simulink model "robot_delta_PID_v3"  (R2024b)
settings: Solver=ode1  StartTime=0  StopTime=10  FixedStep=1e-6  MaxStep=1e-6  RelTol=1e-6
model workspace (MAT data in the model file):
  Ts = 1e-06
  kd1 = 14
  kd2 = 13.6
  kd3 = 37.9
  ki1 = 39
  ki2 = 36
  ki3 = 11.6
  kp1 = 12.6
  kp2 = 12.2
  kp3 = 14.4
undefined symbols (not defined in the file or in its folder): DiscIntNeverNeededParam
libraries: spsUniversalBridgeLib x6, spsCurrentMeasurementLib x6, spsDCVoltageSourceLib x3, spsStepperMotorLib x3, spspowerguiLib x1
settings Model: Creator=rodri  LastModifiedBy=rodri
settings SolverCC: InitialStep=1e-6

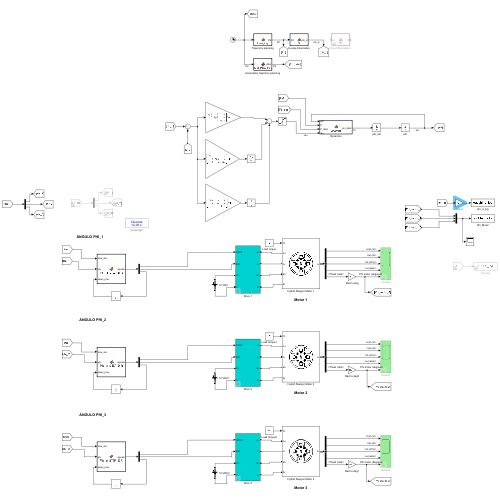
[thumbnail: Simulink's stored preview of the top-level diagram]
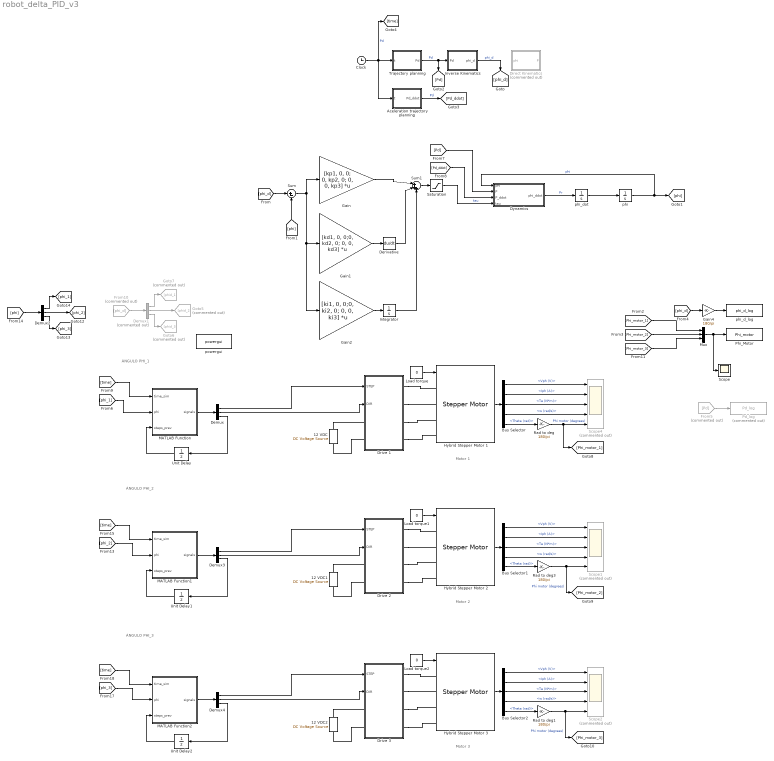
== system robot_delta_PID_v3 ==
  note: Motor 1
  note: ÁNGULO PHI_1
  note: ÁNGULO PHI_2
  note: ÁNGULO PHI_3
  note: Motor 2
  note: Motor 3
  12 VDC : spsDCVoltageSourceLib/DC Voltage Source  Amplitude=12  Measurements=None
  12 VDC1 : spsDCVoltageSourceLib/DC Voltage Source  Amplitude=12  Measurements=None
  12 VDC2 : spsDCVoltageSourceLib/DC Voltage Source  Amplitude=12  Measurements=None
  Aceleration trajectory planning : MATLAB Function  TreatAsAtomicUnit=on
  Bus Selector : BusSelector  OutputSignals=Vph (V),Iph (A),Te (N*m),w (rad/s),Theta (rad)
  Bus Selector1 : BusSelector  OutputSignals=Vph (V),Iph (A),Te (N*m),w (rad/s),Theta (rad)
  Bus Selector2 : BusSelector  OutputSignals=Vph (V),Iph (A),Te (N*m),w (rad/s),Theta (rad)
  Clock : Clock
  Demux{,2..4} (4 alike) : Demux  Outputs=3
  Demux1 : Demux  Commented=on  Outputs=3
  Derivative : Derivative
  Direct Kinematics : MATLAB Function  Commented=on  TreatAsAtomicUnit=on
  Drive 1 : Subsystem  mask{Iref=2, step=500, Ts=Ts}
      mask prompts: Iref "Phase current (A)"; step "Stepping rate (step/s)"; Ts "Sampling time (s)"
      mask init:
      | Nstep=round(1/step/Ts);
  Drive 2 : Subsystem  mask{Iref=2, step=500, Ts=Ts}
      mask prompts: Iref "Phase current (A)"; step "Stepping rate (step/s)"; Ts "Sampling time (s)"
      mask init:
      | Nstep=round(1/step/Ts);
  Drive 3 : Subsystem  mask{Iref=2, step=500, Ts=Ts}
      mask prompts: Iref "Phase current (A)"; step "Stepping rate (step/s)"; Ts "Sampling time (s)"
      mask init:
      | Nstep=round(1/step/Ts);
  Dynamics : MATLAB Function  TreatAsAtomicUnit=on
  From10 : From  Commented=on  GotoTag=phi_d
  From5 : From  Commented=on  GotoTag=Pd
  Gain : Gain  Gain=[kp1, 0, 0; 0, kp2, 0; 0, 0, kp3]  Multiplication=Matrix(K*u)
  Gain1 : Gain  Gain=[kd1, 0, 0;0, kd2, 0; 0, 0, kd3]  Multiplication=Matrix(K*u)
  Gain2 : Gain  Gain=[ki1, 0, 0;0, ki2, 0; 0, 0, ki3]  Multiplication=Matrix(K*u)
  Gain4 : Gain  Gain=180/pi
  Goto5 : Goto  Commented=on  GotoTag=phid_2
  Goto6 : Goto  Commented=on  GotoTag=phid_3
  Goto7 : Goto  Commented=on  GotoTag=phid_1
  Hybrid Stepper Motor 1 : spsStepperMotorLib/Stepper Motor  MotorType=Permanent-magnet / Hybrid  NumberOfPhases_1=2  NumberOfPhases_2=3  PresetModel_1=<empty>  PresetModel_2=<empty>  L=2.8e-3  Lmax=10e-3  Lmin=2e-3  R=1.5  Step_angle=360/1600  Psim=0.005  Tdm=2.2/100  J=54/(1000*100^2)  B=1e-7*1000  w0=0  pos0=0  TsPowergui=0  TsBlock=-1
  Hybrid Stepper Motor 2 : spsStepperMotorLib/Stepper Motor  MotorType=Permanent-magnet / Hybrid  NumberOfPhases_1=2  NumberOfPhases_2=3  PresetModel_1=<empty>  PresetModel_2=<empty>  L=2.8e-3  Lmax=10e-3  Lmin=2e-3  R=1.5  Step_angle=360/1600  Psim=0.005  Tdm=2.2/100  J=54/(1000*100^2)  B=1e-7*1000  w0=0  pos0=0  TsPowergui=0  TsBlock=-1
  Hybrid Stepper Motor 3 : spsStepperMotorLib/Stepper Motor  MotorType=Permanent-magnet / Hybrid  NumberOfPhases_1=2  NumberOfPhases_2=3  PresetModel_1=<empty>  PresetModel_2=<empty>  L=2.8e-3  Lmax=10e-3  Lmin=2e-3  R=1.5  Step_angle=360/1600  Psim=0.005  Tdm=2.2/100  J=54/(1000*100^2)  B=1e-7*1000  w0=0  pos0=0  TsPowergui=0  TsBlock=-1
  Integrator : Integrator  InitialCondition=[0;0;0]
  Inverse Kinematics : MATLAB Function  TreatAsAtomicUnit=on
  Load torque : Constant  Value=0
  Load torque1 : Constant  Value=0
  Load torque2 : Constant  Value=0
  MATLAB Function : MATLAB Function  TreatAsAtomicUnit=on
  MATLAB Function1 : MATLAB Function  TreatAsAtomicUnit=on
  MATLAB Function2 : MATLAB Function  TreatAsAtomicUnit=on
  Mux : Mux  Inputs=3
  Pd_log : ToWorkspace  Commented=on  VariableName=Pd_log  SampleTime=-1
  Phi_Motor : ToWorkspace  VariableName=Phi_motor  SampleTime=-1
  Rad to deg : Gain  Gain=180/pi
  Rad to deg1 : Gain  Gain=180/pi
  Rad to deg3 : Gain  Gain=180/pi
  Saturation : Saturate  UpperLimit=19.8  LowerLimit=-19.8
  Scope : Scope
  Scope1 : Scope  Commented=on  NumInputPorts=5
  Scope2 : Scope  Commented=on  NumInputPorts=5
  Scope4 : Scope  Commented=on  NumInputPorts=5
  Sum : Sum  Inputs=|+-
  Sum1 : Sum  Inputs=|+++
  Trajectory planning : MATLAB Function  TreatAsAtomicUnit=on
  Unit Delay : UnitDelay  SampleTime=-1  HasFrameUpgradeWarning=on
  Unit Delay1 : UnitDelay  SampleTime=-1  HasFrameUpgradeWarning=on
  Unit Delay2 : UnitDelay  SampleTime=-1  HasFrameUpgradeWarning=on
  phi : Integrator  InitialCondition=[0;0;0]
  phi_d_log : ToWorkspace  VariableName=phi_d_log  SampleTime=-1
  phi_dot : Integrator  InitialCondition=[0;0;0]
  powergui : spspowerguiLib/powergui  SimulationMode=Discrete  SampleTime=Ts  frequency=60  Iterations=50  frequencyindice=0  Pbase=100e6  ErrMax=1e-4  UnitsV=kV  UnitsW=MW  buscounter=0  FunctionMessages=off  echomessages=off  EnableUseOfTLC=off  CurrentSourceSwitches=off  DisableSnubberDevices=off  DisableRonSwitches=off  DisableVfSwitches=off  DisplayEquations=off  AutomaticDiscreteSolvers=off  SolverType=Tustin/Backward Euler (TBE)  Interpol=off  ExternalGateDelay=off  methode=off  Ts=0  x0status=blocks  SPID=off  SwTol=0  HookPort=off  NonlinearTolerance=1e-4  nMaxIteration=100  ContinueOnMaxIteration=off  RestoreLinks=warning  ResistiveCurrentMeasurement=off  Frange=[0:2:500]  Ylog=off  Xlog=on  ShowGrid=off  save=off  variable=ZData  structure=0  ZoomFFT=on  StartTime=0.0  cycles=1  DisplayStyle=1  fundamental=60  FreqAxis=off  MaxFrequency=1000  frequencyindicesteady=1  RmsSteady=1  display=off
  wires:
  Trajectory planning/1(Pd) -> Inverse Kinematics/1(Pd), [Pd]  "Pd"
  Inverse Kinematics/1(phi_d) -> [phi_d]  "phi_d"
  Dynamics/1(phi_ddot) -> phi_dot/1  "Pr"
  phi_dot/1 -> phi/1
  phi/1 -> Dynamics/1(phi), [phi]  "phi"
  [phi_d] -> Sum/1
  [phi] -> Sum/2
  Sum/1 -> Gain2/1, Gain1/1, Gain/1
  Gain1/1 -> Derivative/1
  Gain/1 -> Sum1/1
  Derivative/1 -> Sum1/2
  [Pd] -> Dynamics/2(P)
  [Pd_ddot] -> Dynamics/3(P_ddot)
  Clock/1 -> [time], Aceleration trajectory planning/1(t), Trajectory planning/1(t)  "Pd"
  Aceleration trajectory planning/1(Pd_ddot) -> [Pd_ddot]  "Pd"
  Gain2/1 -> Integrator/1
  Integrator/1 -> Sum1/3
  Sum1/1 -> Saturation/1
  Saturation/1 -> Dynamics/4(tau)  "tau"
  From5/1 -> Pd_log/1
  Demux2/2 -> [phi_2]
  Demux2/1 -> [phi_1]
  Demux2/3 -> [phi_3]
  [phi] -> Demux2/1
  [time] -> MATLAB Function/1(time_sim)
  Bus Selector/5 -> Rad to deg/1  "<Theta (rad)>"
  Hybrid Stepper Motor 1/1 -> Bus Selector/1
  Bus Selector/4 -> Scope4/4  "<w (rad/s)>"
  MATLAB Function/1(signals) -> Demux/1
  [phi_1] -> MATLAB Function/2(phi)
  Bus Selector/1 -> Scope4/1  "<Vph (V)>"
  Demux/1 -> Drive 1/1(STEP)
  Demux/2 -> Drive 1/2(DIR)
  Rad to deg/1 -> [Phi_motor_1], Scope4/5  "Phi motor (degrees)"
  Demux/3 -> Unit Delay/1
  Unit Delay/1 -> MATLAB Function/3(steps_prev)
  Bus Selector/2 -> Scope4/2  "<Iph (A)>"
  Bus Selector/3 -> Scope4/3  "<Te (N*m)>"
  Demux1/1 -> Goto7/1
  Demux1/3 -> Goto6/1
  From10/1 -> Demux1/1
  Demux1/2 -> Goto5/1
  Load torque/1 -> Hybrid Stepper Motor 1/1
  MATLAB Function1/1(signals) -> Demux3/1
  Demux3/1 -> Drive 2/1(STEP)
  Load torque1/1 -> Hybrid Stepper Motor 2/1
  Demux3/3 -> Unit Delay1/1
  Hybrid Stepper Motor 2/1 -> Bus Selector1/1
  Unit Delay1/1 -> MATLAB Function1/3(steps_prev)
  [time] -> MATLAB Function1/1(time_sim)
  [phi_2] -> MATLAB Function1/2(phi)
  Demux3/2 -> Drive 2/2(DIR)
  Bus Selector1/3 -> Scope1/3  "<Te (N*m)>"
  Rad to deg3/1 -> [Phi_motor_2], Scope1/5  "Phi motor (degrees)"
  Bus Selector1/4 -> Scope1/4  "<w (rad/s)>"
  Bus Selector1/2 -> Scope1/2  "<Iph (A)>"
  Bus Selector1/5 -> Rad to deg3/1  "<Theta (rad)>"
  Bus Selector1/1 -> Scope1/1  "<Vph (V)>"
  Bus Selector2/1 -> Scope2/1  "<Vph (V)>"
  Bus Selector2/2 -> Scope2/2  "<Iph (A)>"
  Rad to deg1/1 -> [Phi_motor_3], Scope2/5  "Phi motor (degrees)"
  [phi_3] -> MATLAB Function2/2(phi)
  Bus Selector2/3 -> Scope2/3  "<Te (N*m)>"
  Demux4/2 -> Drive 3/2(DIR)
  [time] -> MATLAB Function2/1(time_sim)
  Unit Delay2/1 -> MATLAB Function2/3(steps_prev)
  Hybrid Stepper Motor 3/1 -> Bus Selector2/1
  Demux4/3 -> Unit Delay2/1
  MATLAB Function2/1(signals) -> Demux4/1
  Demux4/1 -> Drive 3/1(STEP)
  Bus Selector2/5 -> Rad to deg1/1  "<Theta (rad)>"
  Bus Selector2/4 -> Scope2/4  "<w (rad/s)>"
  Load torque2/1 -> Hybrid Stepper Motor 3/1
  Mux/1 -> Scope/1, Phi_Motor/1
  Gain4/1 -> phi_d_log/1
  [phi_d] -> Gain4/1
  [Phi_motor_1] -> Mux/1
  [Phi_motor_2] -> Mux/2
  [Phi_motor_3] -> Mux/3
  connections:
  Drive 1/RConn3 -- Hybrid Stepper Motor 1/LConn3
  Drive 1/RConn4 -- Hybrid Stepper Motor 1/LConn4
  Drive 1/RConn2 -- Hybrid Stepper Motor 1/LConn2
  12 VDC/RConn1 -- Drive 1/LConn1
  Drive 1/LConn2 -- 12 VDC/LConn1
  Drive 1/RConn1 -- Hybrid Stepper Motor 1/LConn1
  12 VDC1/RConn1 -- Drive 2/LConn1
  Drive 2/RConn4 -- Hybrid Stepper Motor 2/LConn4
  Drive 2/LConn2 -- 12 VDC1/LConn1
  Drive 2/RConn1 -- Hybrid Stepper Motor 2/LConn1
  Drive 2/RConn2 -- Hybrid Stepper Motor 2/LConn2
  Drive 2/RConn3 -- Hybrid Stepper Motor 2/LConn3
  12 VDC2/RConn1 -- Drive 3/LConn1
  Drive 3/RConn4 -- Hybrid Stepper Motor 3/LConn4
  Drive 3/RConn1 -- Hybrid Stepper Motor 3/LConn1
  Drive 3/LConn2 -- 12 VDC2/LConn1
  Drive 3/RConn3 -- Hybrid Stepper Motor 3/LConn3
  Drive 3/RConn2 -- Hybrid Stepper Motor 3/LConn2

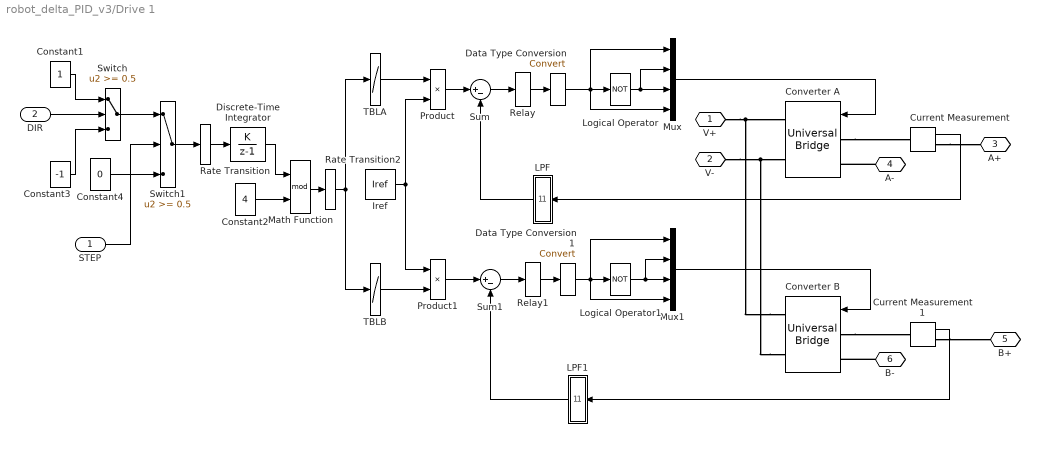
== system robot_delta_PID_v3/Drive 1 ==
  STEP : Inport
  DIR : Inport  Port=2
  Constant1 : Constant  SampleTime=Ts
  Constant2 : Constant  Value=4  SampleTime=Nstep*Ts
  Constant3 : Constant  Value=-1  SampleTime=Ts
  Constant4 : Constant  Value=0  SampleTime=Ts
  Converter A : spsUniversalBridgeLib/Universal Bridge  Arms=2  SnubberResistance=10000  SnubberCapacitance=inf  Device=MOSFET / Diodes  Ron=1e-3*10  Lon=0  ForwardVoltages="[  0  0  ]"  ForwardVoltage=0  GTOparameters=[ 10e-6 , 20e-6 ]  IGBTparameters=[ 0.5e-6 , 0.5e-6 ]  Measurements=None  Measurements_2=None  converterType=Rectifier
  Converter B : spsUniversalBridgeLib/Universal Bridge  Arms=2  SnubberResistance=10000  SnubberCapacitance=inf  Device=MOSFET / Diodes  Ron=1e-3*10  Lon=0  ForwardVoltages="[  0  0  ]"  ForwardVoltage=0  GTOparameters=[ 10e-6 , 20e-6 ]  IGBTparameters=[ 0.5e-6 , 0.5e-6 ]  Measurements=None  Measurements_2=None  converterType=Rectifier
  Current Measurement : spsCurrentMeasurementLib/Current Measurement  PhasorSimulation=off  OutputType=Complex  PSBequivalent=0
  Current Measurement1 : spsCurrentMeasurementLib/Current Measurement  PhasorSimulation=off  OutputType=Complex  PSBequivalent=0
  Data Type Conversion : DataTypeConversion  SaturateOnIntegerOverflow=off  RndMeth=Floor
  Data Type Conversion1 : DataTypeConversion  SaturateOnIntegerOverflow=off  RndMeth=Floor
  Discrete-Time Integrator : DiscreteIntegrator  IntegratorMethod=Accumulation: Forward Euler  SampleTime=Nstep*Ts  ICPrevOutput=DiscIntNeverNeededParam  ICPrevScaledInput=DiscIntNeverNeededParam
  Iref : Constant  Value=Iref  SampleTime=Ts
  LPF : Subsystem  mask{fc=10000, Ts=Ts}
      mask prompts: fc "Cut-off frequency (Hz)"; Ts "Sampling time (s)"
      mask init:
      | % fa=tf(1,[1/2/pi/fc 1]);
      | % fn=c2d(fa,Ts);
      | % [NN,DD]=tfdata(fn,'v')
      | 
      | NN = [ 0,0.0609];
      | DD = [1.0000,-0.9391];
  LPF1 : Subsystem  mask{fc=10000, Ts=Ts}
      mask prompts: fc "Cut-off frequency (Hz)"; Ts "Sampling time (s)"
      mask init:
      | % fa=tf(1,[1/2/pi/fc 1]);
      | % fn=c2d(fa,Ts);
      | % [NN,DD]=tfdata(fn,'v')
      | 
      | NN = [ 0,0.0609];
      | DD = [1.0000,-0.9391];
  Logical Operator : Logic  Operator=NOT  AllPortsSameDT=off  OutDataTypeStr=boolean
  Logical Operator1 : Logic  Operator=NOT  AllPortsSameDT=off  OutDataTypeStr=boolean
  Math Function : Math  Operator=mod  SignedPower=on  SampleTime=Nstep*Ts
  Mux : Mux
  Mux1 : Mux
  Product : Product  RndMeth=Zero
  Product1 : Product  RndMeth=Zero
  Rate Transition : RateTransition
  Rate Transition2 : RateTransition
  Relay : Relay  OnSwitchValue=0.01  OffSwitchValue=-0.01
  Relay1 : Relay  OnSwitchValue=0.01  OffSwitchValue=-0.01  OutDataTypeStr=Inherit: Inherit via back propagation
  Sum : Sum  Inputs=|+-  OutDataTypeStr=Inherit: Same as first input
  Sum1 : Sum  Inputs=|+-  OutDataTypeStr=Inherit: Same as first input
  Switch : Switch  Threshold=0.5  ZeroCross=off  SampleTime=Ts  SaturateOnIntegerOverflow=off  InputSameDT=off
  Switch1 : Switch  Threshold=0.5  ZeroCross=off  SampleTime=Ts  SaturateOnIntegerOverflow=off  InputSameDT=off
  TBLA : Lookup_n-D  NumberOfTableDimensions=1  BreakpointsForDimension1=[0:3]  BreakpointsForDimension2=[0 571.55 685.8 800.15 914.4 1028.8 1143.1 1257.4 1371.7 1486 1600.3 1714.6 1828.9 1943.2 2057.5 2171.8 2286.1 2400.5 2514.7 2629.1 2743.3 2857.7 2971.9 3086.3 3200.5 3314.9 3429.2]  Table=[1 0 -1 0]  InternalRulePriority=Speed  RndMeth=Simplest
  TBLB : Lookup_n-D  NumberOfTableDimensions=1  BreakpointsForDimension1=[0:3]  BreakpointsForDimension2=[0 571.55 685.8 800.15 914.4 1028.8 1143.1 1257.4 1371.7 1486 1600.3 1714.6 1828.9 1943.2 2057.5 2171.8 2286.1 2400.5 2514.7 2629.1 2743.3 2857.7 2971.9 3086.3 3200.5 3314.9 3429.2]  Table=[0 1 0 -1]  InternalRulePriority=Speed  RndMeth=Simplest
  V+ : PMIOPort  Side=Left
  V- : PMIOPort  Port=2  Side=Left
  A+ : PMIOPort  Port=3  Side=Right
  A- : PMIOPort  Port=4  Side=Right
  B+ : PMIOPort  Port=5  Side=Right
  B- : PMIOPort  Port=6  Side=Right
  wires:
  Constant4/1 -> Switch1/3
  Switch1/1 -> Rate Transition/1
  Switch/1 -> Switch1/1
  STEP/1 -> Switch1/2
  DIR/1 -> Switch/2
  Rate Transition2/1 -> TBLB/1, TBLA/1
  Math Function/1 -> Rate Transition2/1
  Product1/1 -> Sum1/1
  Product/1 -> Sum/1
  Rate Transition/1 -> Discrete-Time Integrator/1
  Constant3/1 -> Switch/3
  Constant1/1 -> Switch/1
  Discrete-Time Integrator/1 -> Math Function/1
  Constant2/1 -> Math Function/2
  Iref/1 -> Product1/1, Product/2
  TBLB/1 -> Product1/2
  TBLA/1 -> Product/1
  LPF1/1(O) -> Sum1/2
  LPF/1(O) -> Sum/2
  Data Type Conversion1/1 -> Mux1/4, Mux1/1, Logical Operator1/1
  Data Type Conversion/1 -> Logical Operator/1, Mux/4, Mux/1
  Current Measurement1/1 -> LPF1/1(I)
  Sum1/1 -> Relay1/1
  Mux1/1 -> Converter B/1
  Logical Operator1/1 -> Mux1/2, Mux1/3
  Relay1/1 -> Data Type Conversion1/1
  Mux/1 -> Converter A/1
  Logical Operator/1 -> Mux/2, Mux/3
  Relay/1 -> Data Type Conversion/1
  Current Measurement/1 -> LPF/1(I)
  Sum/1 -> Relay/1
  connections:
  Converter B/RConn2 -- Converter A/RConn2 -- V-/RConn1
  Converter B/RConn1 -- Converter A/RConn1 -- V+/RConn1
  Current Measurement1/RConn1 -- B+/RConn1
  Converter B/LConn1 -- Current Measurement1/LConn1
  Current Measurement/RConn1 -- A+/RConn1
  Converter A/LConn1 -- Current Measurement/LConn1
  B-/RConn1 -- Converter B/LConn2
  A-/RConn1 -- Converter A/LConn2

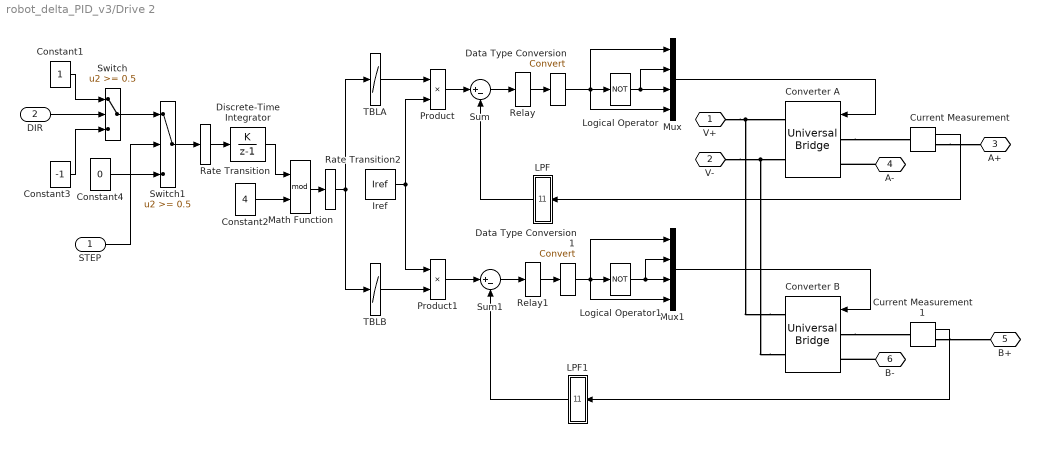
== system robot_delta_PID_v3/Drive 2 ==
  STEP : Inport
  DIR : Inport  Port=2
  Constant1 : Constant  SampleTime=Ts
  Constant2 : Constant  Value=4  SampleTime=Nstep*Ts
  Constant3 : Constant  Value=-1  SampleTime=Ts
  Constant4 : Constant  Value=0  SampleTime=Ts
  Converter A : spsUniversalBridgeLib/Universal Bridge  Arms=2  SnubberResistance=10000  SnubberCapacitance=inf  Device=MOSFET / Diodes  Ron=1e-3*10  Lon=0  ForwardVoltages="[  0  0  ]"  ForwardVoltage=0  GTOparameters=[ 10e-6 , 20e-6 ]  IGBTparameters=[ 0.5e-6 , 0.5e-6 ]  Measurements=None  Measurements_2=None  converterType=Rectifier
  Converter B : spsUniversalBridgeLib/Universal Bridge  Arms=2  SnubberResistance=10000  SnubberCapacitance=inf  Device=MOSFET / Diodes  Ron=1e-3*10  Lon=0  ForwardVoltages="[  0  0  ]"  ForwardVoltage=0  GTOparameters=[ 10e-6 , 20e-6 ]  IGBTparameters=[ 0.5e-6 , 0.5e-6 ]  Measurements=None  Measurements_2=None  converterType=Rectifier
  Current Measurement : spsCurrentMeasurementLib/Current Measurement  PhasorSimulation=off  OutputType=Complex  PSBequivalent=0
  Current Measurement1 : spsCurrentMeasurementLib/Current Measurement  PhasorSimulation=off  OutputType=Complex  PSBequivalent=0
  Data Type Conversion : DataTypeConversion  SaturateOnIntegerOverflow=off  RndMeth=Floor
  Data Type Conversion1 : DataTypeConversion  SaturateOnIntegerOverflow=off  RndMeth=Floor
  Discrete-Time Integrator : DiscreteIntegrator  IntegratorMethod=Accumulation: Forward Euler  SampleTime=Nstep*Ts  ICPrevOutput=DiscIntNeverNeededParam  ICPrevScaledInput=DiscIntNeverNeededParam
  Iref : Constant  Value=Iref  SampleTime=Ts
  LPF : Subsystem  mask{fc=10000, Ts=Ts}
      mask prompts: fc "Cut-off frequency (Hz)"; Ts "Sampling time (s)"
      mask init:
      | % fa=tf(1,[1/2/pi/fc 1]);
      | % fn=c2d(fa,Ts);
      | % [NN,DD]=tfdata(fn,'v')
      | 
      | NN = [ 0,0.0609];
      | DD = [1.0000,-0.9391];
  LPF1 : Subsystem  mask{fc=10000, Ts=Ts}
      mask prompts: fc "Cut-off frequency (Hz)"; Ts "Sampling time (s)"
      mask init:
      | % fa=tf(1,[1/2/pi/fc 1]);
      | % fn=c2d(fa,Ts);
      | % [NN,DD]=tfdata(fn,'v')
      | 
      | NN = [ 0,0.0609];
      | DD = [1.0000,-0.9391];
  Logical Operator : Logic  Operator=NOT  AllPortsSameDT=off  OutDataTypeStr=boolean
  Logical Operator1 : Logic  Operator=NOT  AllPortsSameDT=off  OutDataTypeStr=boolean
  Math Function : Math  Operator=mod  SignedPower=on  SampleTime=Nstep*Ts
  Mux : Mux
  Mux1 : Mux
  Product : Product  RndMeth=Zero
  Product1 : Product  RndMeth=Zero
  Rate Transition : RateTransition
  Rate Transition2 : RateTransition
  Relay : Relay  OnSwitchValue=0.01  OffSwitchValue=-0.01
  Relay1 : Relay  OnSwitchValue=0.01  OffSwitchValue=-0.01  OutDataTypeStr=Inherit: Inherit via back propagation
  Sum : Sum  Inputs=|+-  OutDataTypeStr=Inherit: Same as first input
  Sum1 : Sum  Inputs=|+-  OutDataTypeStr=Inherit: Same as first input
  Switch : Switch  Threshold=0.5  ZeroCross=off  SampleTime=Ts  SaturateOnIntegerOverflow=off  InputSameDT=off
  Switch1 : Switch  Threshold=0.5  ZeroCross=off  SampleTime=Ts  SaturateOnIntegerOverflow=off  InputSameDT=off
  TBLA : Lookup_n-D  NumberOfTableDimensions=1  BreakpointsForDimension1=[0:3]  BreakpointsForDimension2=[0 571.55 685.8 800.15 914.4 1028.8 1143.1 1257.4 1371.7 1486 1600.3 1714.6 1828.9 1943.2 2057.5 2171.8 2286.1 2400.5 2514.7 2629.1 2743.3 2857.7 2971.9 3086.3 3200.5 3314.9 3429.2]  Table=[1 0 -1 0]  InternalRulePriority=Speed  RndMeth=Simplest
  TBLB : Lookup_n-D  NumberOfTableDimensions=1  BreakpointsForDimension1=[0:3]  BreakpointsForDimension2=[0 571.55 685.8 800.15 914.4 1028.8 1143.1 1257.4 1371.7 1486 1600.3 1714.6 1828.9 1943.2 2057.5 2171.8 2286.1 2400.5 2514.7 2629.1 2743.3 2857.7 2971.9 3086.3 3200.5 3314.9 3429.2]  Table=[0 1 0 -1]  InternalRulePriority=Speed  RndMeth=Simplest
  V+ : PMIOPort  Side=Left
  V- : PMIOPort  Port=2  Side=Left
  A+ : PMIOPort  Port=3  Side=Right
  A- : PMIOPort  Port=4  Side=Right
  B+ : PMIOPort  Port=5  Side=Right
  B- : PMIOPort  Port=6  Side=Right
  wires:
  Constant4/1 -> Switch1/3
  Switch1/1 -> Rate Transition/1
  Switch/1 -> Switch1/1
  STEP/1 -> Switch1/2
  DIR/1 -> Switch/2
  Rate Transition2/1 -> TBLB/1, TBLA/1
  Math Function/1 -> Rate Transition2/1
  Product1/1 -> Sum1/1
  Product/1 -> Sum/1
  Rate Transition/1 -> Discrete-Time Integrator/1
  Constant3/1 -> Switch/3
  Constant1/1 -> Switch/1
  Discrete-Time Integrator/1 -> Math Function/1
  Constant2/1 -> Math Function/2
  Iref/1 -> Product1/1, Product/2
  TBLB/1 -> Product1/2
  TBLA/1 -> Product/1
  LPF1/1(O) -> Sum1/2
  LPF/1(O) -> Sum/2
  Data Type Conversion1/1 -> Mux1/4, Mux1/1, Logical Operator1/1
  Data Type Conversion/1 -> Logical Operator/1, Mux/4, Mux/1
  Current Measurement1/1 -> LPF1/1(I)
  Sum1/1 -> Relay1/1
  Mux1/1 -> Converter B/1
  Logical Operator1/1 -> Mux1/2, Mux1/3
  Relay1/1 -> Data Type Conversion1/1
  Mux/1 -> Converter A/1
  Logical Operator/1 -> Mux/2, Mux/3
  Relay/1 -> Data Type Conversion/1
  Current Measurement/1 -> LPF/1(I)
  Sum/1 -> Relay/1
  connections:
  Converter B/RConn2 -- Converter A/RConn2 -- V-/RConn1
  Converter B/RConn1 -- Converter A/RConn1 -- V+/RConn1
  Current Measurement1/RConn1 -- B+/RConn1
  Converter B/LConn1 -- Current Measurement1/LConn1
  Current Measurement/RConn1 -- A+/RConn1
  Converter A/LConn1 -- Current Measurement/LConn1
  B-/RConn1 -- Converter B/LConn2
  A-/RConn1 -- Converter A/LConn2

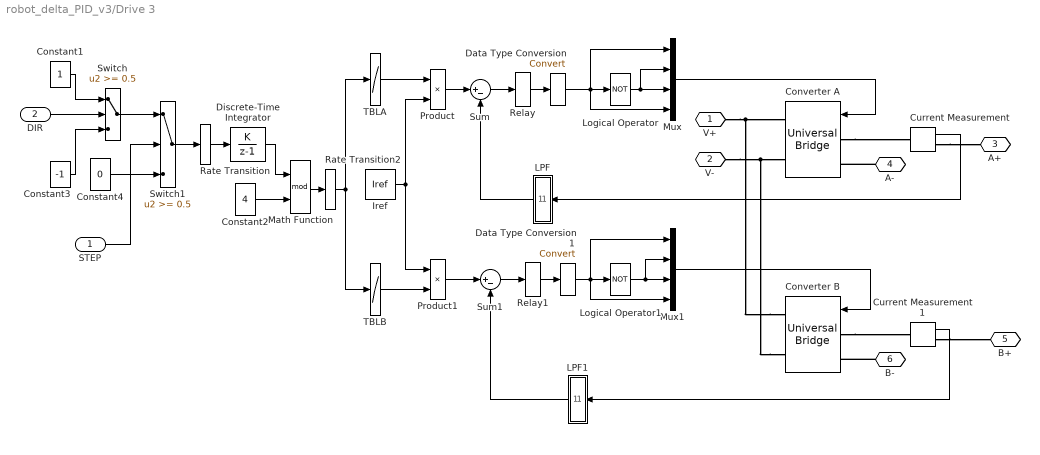
== system robot_delta_PID_v3/Drive 3 ==
  STEP : Inport
  DIR : Inport  Port=2
  Constant1 : Constant  SampleTime=Ts
  Constant2 : Constant  Value=4  SampleTime=Nstep*Ts
  Constant3 : Constant  Value=-1  SampleTime=Ts
  Constant4 : Constant  Value=0  SampleTime=Ts
  Converter A : spsUniversalBridgeLib/Universal Bridge  Arms=2  SnubberResistance=10000  SnubberCapacitance=inf  Device=MOSFET / Diodes  Ron=1e-3*10  Lon=0  ForwardVoltages="[  0  0  ]"  ForwardVoltage=0  GTOparameters=[ 10e-6 , 20e-6 ]  IGBTparameters=[ 0.5e-6 , 0.5e-6 ]  Measurements=None  Measurements_2=None  converterType=Rectifier
  Converter B : spsUniversalBridgeLib/Universal Bridge  Arms=2  SnubberResistance=10000  SnubberCapacitance=inf  Device=MOSFET / Diodes  Ron=1e-3*10  Lon=0  ForwardVoltages="[  0  0  ]"  ForwardVoltage=0  GTOparameters=[ 10e-6 , 20e-6 ]  IGBTparameters=[ 0.5e-6 , 0.5e-6 ]  Measurements=None  Measurements_2=None  converterType=Rectifier
  Current Measurement : spsCurrentMeasurementLib/Current Measurement  PhasorSimulation=off  OutputType=Complex  PSBequivalent=0
  Current Measurement1 : spsCurrentMeasurementLib/Current Measurement  PhasorSimulation=off  OutputType=Complex  PSBequivalent=0
  Data Type Conversion : DataTypeConversion  SaturateOnIntegerOverflow=off  RndMeth=Floor
  Data Type Conversion1 : DataTypeConversion  SaturateOnIntegerOverflow=off  RndMeth=Floor
  Discrete-Time Integrator : DiscreteIntegrator  IntegratorMethod=Accumulation: Forward Euler  SampleTime=Nstep*Ts  ICPrevOutput=DiscIntNeverNeededParam  ICPrevScaledInput=DiscIntNeverNeededParam
  Iref : Constant  Value=Iref  SampleTime=Ts
  LPF : Subsystem  mask{fc=10000, Ts=Ts}
      mask prompts: fc "Cut-off frequency (Hz)"; Ts "Sampling time (s)"
      mask init:
      | % fa=tf(1,[1/2/pi/fc 1]);
      | % fn=c2d(fa,Ts);
      | % [NN,DD]=tfdata(fn,'v')
      | 
      | NN = [ 0,0.0609];
      | DD = [1.0000,-0.9391];
  LPF1 : Subsystem  mask{fc=10000, Ts=Ts}
      mask prompts: fc "Cut-off frequency (Hz)"; Ts "Sampling time (s)"
      mask init:
      | % fa=tf(1,[1/2/pi/fc 1]);
      | % fn=c2d(fa,Ts);
      | % [NN,DD]=tfdata(fn,'v')
      | 
      | NN = [ 0,0.0609];
      | DD = [1.0000,-0.9391];
  Logical Operator : Logic  Operator=NOT  AllPortsSameDT=off  OutDataTypeStr=boolean
  Logical Operator1 : Logic  Operator=NOT  AllPortsSameDT=off  OutDataTypeStr=boolean
  Math Function : Math  Operator=mod  SignedPower=on  SampleTime=Nstep*Ts
  Mux : Mux
  Mux1 : Mux
  Product : Product  RndMeth=Zero
  Product1 : Product  RndMeth=Zero
  Rate Transition : RateTransition
  Rate Transition2 : RateTransition
  Relay : Relay  OnSwitchValue=0.01  OffSwitchValue=-0.01
  Relay1 : Relay  OnSwitchValue=0.01  OffSwitchValue=-0.01  OutDataTypeStr=Inherit: Inherit via back propagation
  Sum : Sum  Inputs=|+-  OutDataTypeStr=Inherit: Same as first input
  Sum1 : Sum  Inputs=|+-  OutDataTypeStr=Inherit: Same as first input
  Switch : Switch  Threshold=0.5  ZeroCross=off  SampleTime=Ts  SaturateOnIntegerOverflow=off  InputSameDT=off
  Switch1 : Switch  Threshold=0.5  ZeroCross=off  SampleTime=Ts  SaturateOnIntegerOverflow=off  InputSameDT=off
  TBLA : Lookup_n-D  NumberOfTableDimensions=1  BreakpointsForDimension1=[0:3]  BreakpointsForDimension2=[0 571.55 685.8 800.15 914.4 1028.8 1143.1 1257.4 1371.7 1486 1600.3 1714.6 1828.9 1943.2 2057.5 2171.8 2286.1 2400.5 2514.7 2629.1 2743.3 2857.7 2971.9 3086.3 3200.5 3314.9 3429.2]  Table=[1 0 -1 0]  InternalRulePriority=Speed  RndMeth=Simplest
  TBLB : Lookup_n-D  NumberOfTableDimensions=1  BreakpointsForDimension1=[0:3]  BreakpointsForDimension2=[0 571.55 685.8 800.15 914.4 1028.8 1143.1 1257.4 1371.7 1486 1600.3 1714.6 1828.9 1943.2 2057.5 2171.8 2286.1 2400.5 2514.7 2629.1 2743.3 2857.7 2971.9 3086.3 3200.5 3314.9 3429.2]  Table=[0 1 0 -1]  InternalRulePriority=Speed  RndMeth=Simplest
  V+ : PMIOPort  Side=Left
  V- : PMIOPort  Port=2  Side=Left
  A+ : PMIOPort  Port=3  Side=Right
  A- : PMIOPort  Port=4  Side=Right
  B+ : PMIOPort  Port=5  Side=Right
  B- : PMIOPort  Port=6  Side=Right
  wires:
  Constant4/1 -> Switch1/3
  Switch1/1 -> Rate Transition/1
  Switch/1 -> Switch1/1
  STEP/1 -> Switch1/2
  DIR/1 -> Switch/2
  Rate Transition2/1 -> TBLB/1, TBLA/1
  Math Function/1 -> Rate Transition2/1
  Product1/1 -> Sum1/1
  Product/1 -> Sum/1
  Rate Transition/1 -> Discrete-Time Integrator/1
  Constant3/1 -> Switch/3
  Constant1/1 -> Switch/1
  Discrete-Time Integrator/1 -> Math Function/1
  Constant2/1 -> Math Function/2
  Iref/1 -> Product1/1, Product/2
  TBLB/1 -> Product1/2
  TBLA/1 -> Product/1
  LPF1/1(O) -> Sum1/2
  LPF/1(O) -> Sum/2
  Data Type Conversion1/1 -> Mux1/4, Mux1/1, Logical Operator1/1
  Data Type Conversion/1 -> Logical Operator/1, Mux/4, Mux/1
  Current Measurement1/1 -> LPF1/1(I)
  Sum1/1 -> Relay1/1
  Mux1/1 -> Converter B/1
  Logical Operator1/1 -> Mux1/2, Mux1/3
  Relay1/1 -> Data Type Conversion1/1
  Mux/1 -> Converter A/1
  Logical Operator/1 -> Mux/2, Mux/3
  Relay/1 -> Data Type Conversion/1
  Current Measurement/1 -> LPF/1(I)
  Sum/1 -> Relay/1
  connections:
  Converter B/RConn2 -- Converter A/RConn2 -- V-/RConn1
  Converter B/RConn1 -- Converter A/RConn1 -- V+/RConn1
  Current Measurement1/RConn1 -- B+/RConn1
  Converter B/LConn1 -- Current Measurement1/LConn1
  Current Measurement/RConn1 -- A+/RConn1
  Converter A/LConn1 -- Current Measurement/LConn1
  B-/RConn1 -- Converter B/LConn2
  A-/RConn1 -- Converter A/LConn2

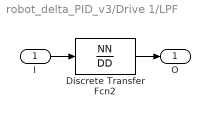
== system robot_delta_PID_v3/Drive 1/LPF ==
  I : Inport
  Discrete Transfer Fcn2 : DiscreteTransferFcn  Numerator=NN  Denominator=DD  SampleTime=Ts
  O : Outport  VectorParamsAs1DForOutWhenUnconnected=off
  wires:
  Discrete Transfer Fcn2/1 -> O/1
  I/1 -> Discrete Transfer Fcn2/1

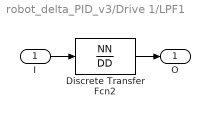
== system robot_delta_PID_v3/Drive 1/LPF1 ==
  I : Inport
  Discrete Transfer Fcn2 : DiscreteTransferFcn  Numerator=NN  Denominator=DD  SampleTime=Ts
  O : Outport  VectorParamsAs1DForOutWhenUnconnected=off
  wires:
  I/1 -> Discrete Transfer Fcn2/1
  Discrete Transfer Fcn2/1 -> O/1

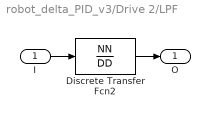
== system robot_delta_PID_v3/Drive 2/LPF ==
  I : Inport
  Discrete Transfer Fcn2 : DiscreteTransferFcn  Numerator=NN  Denominator=DD  SampleTime=Ts
  O : Outport  VectorParamsAs1DForOutWhenUnconnected=off
  wires:
  Discrete Transfer Fcn2/1 -> O/1
  I/1 -> Discrete Transfer Fcn2/1

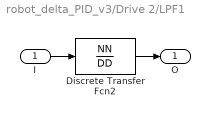
== system robot_delta_PID_v3/Drive 2/LPF1 ==
  I : Inport
  Discrete Transfer Fcn2 : DiscreteTransferFcn  Numerator=NN  Denominator=DD  SampleTime=Ts
  O : Outport  VectorParamsAs1DForOutWhenUnconnected=off
  wires:
  I/1 -> Discrete Transfer Fcn2/1
  Discrete Transfer Fcn2/1 -> O/1

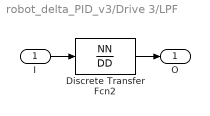
== system robot_delta_PID_v3/Drive 3/LPF ==
  I : Inport
  Discrete Transfer Fcn2 : DiscreteTransferFcn  Numerator=NN  Denominator=DD  SampleTime=Ts
  O : Outport  VectorParamsAs1DForOutWhenUnconnected=off
  wires:
  Discrete Transfer Fcn2/1 -> O/1
  I/1 -> Discrete Transfer Fcn2/1

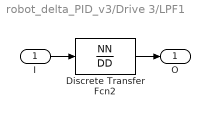
== system robot_delta_PID_v3/Drive 3/LPF1 ==
  I : Inport
  Discrete Transfer Fcn2 : DiscreteTransferFcn  Numerator=NN  Denominator=DD  SampleTime=Ts
  O : Outport  VectorParamsAs1DForOutWhenUnconnected=off
  wires:
  I/1 -> Discrete Transfer Fcn2/1
  Discrete Transfer Fcn2/1 -> O/1

== matlab function robot_delta_PID_v3/Inverse Kinematics ==
  data: Pd input; phi_d output
function phi_d = CI(Pd)
%%%%%%%%%%%%%%%%%%%%%%%%%%
    Xp=Pd(1);
    Yp=Pd(2);
    Zp=Pd(3);
    %%%%%%%%%%%%%%%%%%%%%%%%%%
    % constantes
    L1 = 0.17;
    L2 = 0.32513;
    ra = 0.1;
    rb = 0.0501;
    r = ra - rb;
    theta = [0; 2*pi/3; -2*pi/3]; 

    E = 2*L1*(r - Xp*cos(theta) - Yp*sin(theta));
    F = -2*L1*Zp*[1;1;1];
    G = Xp^2 + Yp^2 + Zp^2 + r^2 + L1^2 - L2^2 - 2*r*(Xp*cos(theta) + Yp*sin(theta));
    sqrt_val = E.^2 + F.^2 - G.^2;
    phi_d = 2*atan((-F - sqrt(sqrt_val))./( G - E));
end

== matlab function robot_delta_PID_v3/Direct Kinematics ==
  data: phi input; P output
function P=CD(phi)
     % Constantes 
    L1 = 0.17;
    L2 = 0.32513;
    ra = 0.1;
    rb = 0.0501;
    r = ra - rb;
    theta = [0; 2*pi/3; -2*pi/3]; 

    % Posiciones de las articulaciones pasivas
    X=(r+L1*cos(phi)).*cos(theta);
    Y=(r+L1*cos(phi)).*sin(theta);
    Z=L1*sin(phi);

    if abs(Z(3)-Z(1))<1e-4 && abs(Z(2)-Z(1))<1e-4
        
        % Definimos matriz del sistema de ecuaciones
        M=[2*(X(3)-X(1)),2*(Y(3)-Y(1));
           2*(X(2)-X(1)),2*(Y(2)-Y(1))];
        b=[X(3)^2+Y(3)^2-(X(1)^2+Y(1)^2);
           X(2)^2+Y(2)^2-(X(1)^2+Y(1)^2)];
        w=M\b;
        Xc=w(1);
        Yc=w(2);
        % Calculamos Z
        Zc=Z(1)+sqrt(L2^2-(Xc-X(1))^2-(Yc-Y(1))^2);
        % Guardamos la solución
        P=[Xc;Yc;Zc];

    elseif abs(X(2)-X(3))<1e-5 && abs(Z(3)-Z(2))<1e-5 && abs(X(3)-X(1))>1e-5 && abs(Z(3)-Z(1))>1e-5

        a=-(Z(3)-Z(1))/(X(3)-X(1)); b=(X(3)^2-X(1)^2+Y(3)^2-Y(1)^2+Z(3)^2-Z(1)^2)/(2*(X(3)-X(1)));
        A=a^2+1; B=2*a*(b-X(3))-2*Z(3); C=(b-X(3))^2+Y(3)^2-L2^2+Z(3)^2;
        Zmas=(-B+sqrt(B^2-4*A*C))/(2*A);
        Xmas=a*Zmas+b;
        Ymas=0;
        P=[Xmas;Ymas;Zmas];
        
    else
        % Definimos coeficientes auxiliares
        a11=2*(X(3)-X(1)); a21=2*(X(3)-X(2));
        a12=2*(Y(3)-Y(1)); a22=2*(Y(3)-Y(2));
        a13=2*(Z(3)-Z(1)); a23=2*(Z(3)-Z(2));

        b1=X(3)^2+Y(3)^2+Z(3)^2-(X(1)^2+Y(1)^2+Z(1)^2);
        b2=X(3)^2+Y(3)^2+Z(3)^2-(X(2)^2+Y(2)^2+Z(2)^2);

        a1=a11/a13-a21/a23; a2=a12/a13-a22/a23; a3=b2/a23-b1/a13;
        a4=-a2/a1; a5=-a3/a1;
        a6=-(a21*a4+a22)/a23; a7=(b2-a21*a5)/a23;

        A=a4^2+1+a6^2;
        B=2*a4*(a5-X(1))-2*Y(1)+2*a6*(a7-Z(1));
        C=a5*(a5-2*X(1))+a7*(a7-2*Z(1))+X(1)^2+Y(1)^2+Z(1)^2-L2^2;

        % Calculamos las dos posibles soluciones
        Ymas=(-B+sqrt(B^2-4*A*C))/(2*A); Xmas=a4*Ymas+a5; Zmas=a6*Ymas+a7;
        Ymenos=(-B-sqrt(B^2-4*A*C))/(2*A); Xmenos=a4*Ymenos+a5; Zmenos=a6*Ymenos+a7;
        
        % Guardamos la solución correcta
        if Zmas>0
            P=[Xmas;Ymas;Zmas]; 
        else
            P=[Xmenos;Ymenos;Zmenos];
        end
    end
end

== matlab function robot_delta_PID_v3/Trajectory planning ==
  data: t input; Pd output
function Pd = Plan_tray(t)
        %% Descripción
        %% Parámetros
        r=0.15; %0.1
        h=0; %0.3;
        k=0; %0.3;
        %% Ecuaciones
        xd=r*cos(t)+h;
        yd=r*sin(t)+k;
        zd=0.23;
        Pd=[xd; yd; zd];
    end

== matlab function robot_delta_PID_v3/Dynamics ==
  data: phi input; P input; P_ddot input; tau input; phi_ddot output
function phi_ddot=Dinamica(phi,P,P_ddot,tau)
    % Constantes
    L1 = 0.17;
    L2 = 0.32513;
    ra = 0.1;
    rb = 0.0501;
    r = ra - rb;
    mp=0.2;
    m1=0.103;
    m2=0.124;
    Im=0.01;
    g=9.81;
    Fpx=0;
    Fpy=0;
    Fpz=0;
    theta = [0; 2*pi/3; -2*pi/3];
    G=[0;0;g];
    Fext=[Fpx;Fpy;Fpz];

    % Constantes auxiliares
    Mpos=(mp+3*m2)/2;
    Mphi=m1/2+m2;
    I=Im+m1*L1^2/3+m2*L1^2;
    
    % Posición del efector final
    Xp=P(1);
    Yp=P(2);
    Zp=P(3);
    
    % Posiciones de las articulaciones pasivas
    X=(r+L1*cos(phi)).*cos(theta);
    Y=(r+L1*cos(phi)).*sin(theta);
    Z=L1*sin(phi);

    % Se definen matrices y vectores para el sistema de ecuaciones
    %de las variables de posición 
    A=[Xp-X(1),Xp-X(2),Xp-X(3);
       Yp-Y(1),Yp-Y(2),Yp-Y(3);
       Zp-Z(1),Zp-Z(2),Zp-Z(3)];
    Lambda=A\(Mpos*(P_ddot+G)-0.5*Fext);
    
    % Se definen matrices y vectores para el sistema de ecuaciones
    %de las variables de phi_1i
    B=2*L1*((-r+Xp*cos(theta)+Yp*sin(theta)).*sin(phi)-Zp*cos(phi));
    phi_ddot=(tau-Mphi*g*L1*cos(phi)+B.*Lambda)/I;
end

== matlab function robot_delta_PID_v3/Aceleration trajectory planning ==
  data: t input; Pd_ddot output
function Pd_ddot = Acel_Plan_tray(t)
        %% Descripción
        %% Parámetros
        r=0.15; %0.1
        %% Ecuaciones
        xd_ddot=-r*cos(t);
        yd_ddot=-r*sin(t);
        zd_ddot=0;
        Pd_ddot=[xd_ddot; yd_ddot; zd_ddot];
    end

== matlab function robot_delta_PID_v3/MATLAB Function ==
  data: time_sim input; phi input; steps_prev input; signals output
function signals = Phi_to_STEP_DIR(time_sim,phi,steps_prev)
    max_steps_per_second=500; % Número máximo de pasos por segundo que puede dar el motor.
    Ts=1e-6; %Periodo de muestreo.
    iterations_per_step = round((1/Ts) / max_steps_per_second);
    t=round(time_sim / Ts);
    if iterations_per_step < 1
        iterations_per_step = 1; % Debe esperar al menos 1 ciclo
    end

    % Esta función controla la velocidad usando un intervalo de iteraciones ('iterations_per_step').
    
    % --- Constantes del motor ---
    deg_per_step = 360/1600;%1.8;
    
    % --- Lógica de control ---
    % 1. Convertir ángulo objetivo a pasos objetivo
    steps_target = floor(rad2deg(phi) / deg_per_step);

    % 2. Determinar la dirección del movimiento
    if steps_target > steps_prev
        DIR = 1; % Dirección positiva
    elseif steps_target < steps_prev
        DIR = 0; % Dirección negativa
    else
        DIR = 0; % Ya estamos en el objetivo, la dirección no importa
    end

    % 3. Decidir si generar un pulso STEP en este ciclo de tiempo
    STEP = 0; % Por defecto, no se genera pulso
    
    % Condición para dar un paso:
    % a) No hemos llegado al objetivo (steps_target ~= steps_prev)
    % b) Ha pasado el número de iteraciones requerido (mod(t, iterations_per_step) == 0)
    if (steps_target ~= steps_prev) && (mod(t, iterations_per_step) == 0)
        STEP = 1; % Generar el pulso
        
        % Actualizar la posición en pasos según la dirección
        if DIR == 1
            steps_prev = steps_prev + 1;
        else
            steps_prev = steps_prev - 1;
        end
    end
    
    % 4. Devolver las señales calculadas
    signals=[STEP; DIR; steps_prev];
end

== matlab function robot_delta_PID_v3/MATLAB Function1 ==
  data: time_sim input; phi input; steps_prev input; signals output
function signals = Phi_to_STEP_DIR(time_sim,phi,steps_prev)
    max_steps_per_second=500; % Número máximo de pasos por segundo que puede dar el motor.
    Ts=1e-6; %Periodo de muestreo.
    iterations_per_step = round((1/Ts) / max_steps_per_second);
    t=round(time_sim / Ts);
    if iterations_per_step < 1
        iterations_per_step = 1; % Debe esperar al menos 1 ciclo
    end

    % Esta función controla la velocidad usando un intervalo de iteraciones ('iterations_per_step').
    
    % --- Constantes del motor ---
    deg_per_step = 360/1600;%1.8;
    
    % --- Lógica de control ---
    % 1. Convertir ángulo objetivo a pasos objetivo
    steps_target = floor(rad2deg(phi) / deg_per_step);

    % 2. Determinar la dirección del movimiento
    if steps_target > steps_prev
        DIR = 1; % Dirección positiva
    elseif steps_target < steps_prev
        DIR = 0; % Dirección negativa
    else
        DIR = 0; % Ya estamos en el objetivo, la dirección no importa
    end

    % 3. Decidir si generar un pulso STEP en este ciclo de tiempo
    STEP = 0; % Por defecto, no se genera pulso
    
    % Condición para dar un paso:
    % a) No hemos llegado al objetivo (steps_target ~= steps_prev)
    % b) Ha pasado el número de iteraciones requerido (mod(t, iterations_per_step) == 0)
    if (steps_target ~= steps_prev) && (mod(t, iterations_per_step) == 0)
        STEP = 1; % Generar el pulso
        
        % Actualizar la posición en pasos según la dirección
        if DIR == 1
            steps_prev = steps_prev + 1;
        else
            steps_prev = steps_prev - 1;
        end
    end
    
    % 4. Devolver las señales calculadas
    signals=[STEP; DIR; steps_prev];
end

== matlab function robot_delta_PID_v3/MATLAB Function2 ==
  data: time_sim input; phi input; steps_prev input; signals output
function signals = Phi_to_STEP_DIR(time_sim,phi,steps_prev)
    max_steps_per_second=500; % Número máximo de pasos por segundo que puede dar el motor.
    Ts=1e-6; %Periodo de muestreo.
    iterations_per_step = round((1/Ts) / max_steps_per_second);
    t=round(time_sim / Ts);
    if iterations_per_step < 1
        iterations_per_step = 1; % Debe esperar al menos 1 ciclo
    end

    % Esta función controla la velocidad usando un intervalo de iteraciones ('iterations_per_step').
    
    % --- Constantes del motor ---
    deg_per_step = 360/1600;%1.8;
    
    % --- Lógica de control ---
    % 1. Convertir ángulo objetivo a pasos objetivo
    steps_target = floor(rad2deg(phi) / deg_per_step);

    % 2. Determinar la dirección del movimiento
    if steps_target > steps_prev
        DIR = 1; % Dirección positiva
    elseif steps_target < steps_prev
        DIR = 0; % Dirección negativa
    else
        DIR = 0; % Ya estamos en el objetivo, la dirección no importa
    end

    % 3. Decidir si generar un pulso STEP en este ciclo de tiempo
    STEP = 0; % Por defecto, no se genera pulso
    
    % Condición para dar un paso:
    % a) No hemos llegado al objetivo (steps_target ~= steps_prev)
    % b) Ha pasado el número de iteraciones requerido (mod(t, iterations_per_step) == 0)
    if (steps_target ~= steps_prev) && (mod(t, iterations_per_step) == 0)
        STEP = 1; % Generar el pulso
        
        % Actualizar la posición en pasos según la dirección
        if DIR == 1
            steps_prev = steps_prev + 1;
        else
            steps_prev = steps_prev - 1;
        end
    end
    
    % 4. Devolver las señales calculadas
    signals=[STEP; DIR; steps_prev];
end
